simulink model "rcsimulation"  (R2019a)
settings: Solver=VariableStepAuto  StartTime=0.0  StopTime=10.0  RelTol=1e-3
values from neighbouring files (symbols this model uses):
  c = 1e-6    (= 1e-06)    [rc_script_file.m]
  R = 1    [rc_script_file.m]
settings Model: Creator=MahMoud  LastModifiedBy=MahMoud

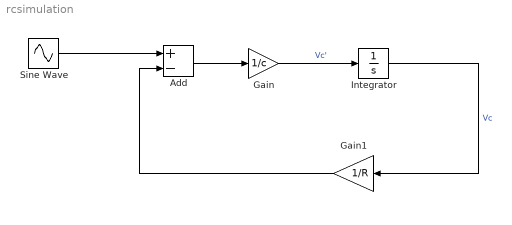
== system rcsimulation ==
  Add : Sum  Inputs=+-
  Gain : Gain  Gain=1/c
  Gain1 : Gain  Gain=1/R
  Integrator : Integrator
  Sine Wave : Sin  Amplitude=5  Frequency=2*pi  SampleTime=0
  wires:
  Gain/1 -> Integrator/1  "Vc'"
  Integrator/1 -> Gain1/1  "Vc"
  Gain1/1 -> Add/2
  Sine Wave/1 -> Add/1
  Add/1 -> Gain/1
